simulink model "Q_4"  (Simulink 10.0)
settings: Solver=VariableStepAuto  StartTime=0.0  StopTime=10.0  RelTol=1e-3
settings Model: Creator=amirhosein  LastModifiedBy=amirhosein
settings DataIOCC: SaveFormat=Dataset  ReturnWorkspaceOutputs=on
settings OptimizationCC: LifeSpan=auto
settings DebuggingCC: UnderspecifiedInitializationDetection=Simplified  MergeDetectMultiDrivingBlocksExec=error  SFUnexpectedBacktrackingDiag=error  SFNoUnconditionalDefaultTransitionDiag=error  SFExecutionAtInitializationDiag=warning  ArithmeticOperatorsInVariantConditions=error
settings HardwareCC: ProdBitPerPointer=64  ProdBitPerSizeT=64  ProdBitPerPtrDiffT=64  ProdLargestAtomicFloat=Float  ProdIntDivRoundTo=Zero  ProdEndianess=LittleEndian  ProdWordSize=64  ProdHWDeviceType=Intel->x86-64 (Windows64)
settings ModelReferenceCC: PropagateSignalLabelsOutOfModel=on
settings SFSimCC: SimUseLocalCustomCode=on  CustomCodeUndefinedFunction=FilterOut
settings RTWCC: RTWUseLocalCustomCode=on
settings CodeAppCC: StateflowObjectComments=off
settings GRTTargetCC: TargetLangStandard=C99 (ISO)  CombineOutputUpdateFcns=on  GRTInterface=off
settings ConfigComp: CovMetricSettings=dwe  CovHtmlReporting=off  CovSaveCumulativeToWorkspaceVar=off  CovSaveSingleToWorkspaceVar=off

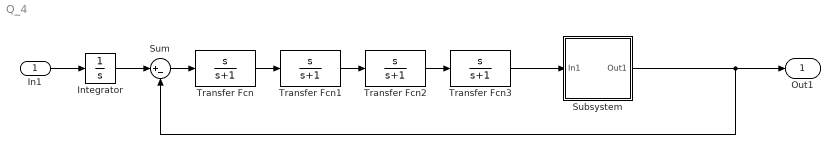
== system Q_4 ==
  In1 : Inport
  Integrator : Integrator
  Subsystem : Subsystem
  Sum : Sum  Inputs=|+-
  Transfer Fcn{,1..3} (4 alike) : TransferFcn  Numerator=[1 0]  Denominator=[1 1]
  Out1 : Outport
  wires:
  Integrator/1 -> Sum/1
  Transfer Fcn1/1 -> Transfer Fcn2/1
  Transfer Fcn/1 -> Transfer Fcn1/1
  Transfer Fcn2/1 -> Transfer Fcn3/1
  Sum/1 -> Transfer Fcn/1
  In1/1 -> Integrator/1
  Subsystem/1(Out1) -> Out1/1, Sum/2
  Transfer Fcn3/1 -> Subsystem/1(In1)

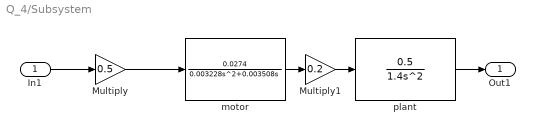
== system Q_4/Subsystem ==
  In1 : Inport
  Multiply : Gain  Gain=0.5
  Multiply1 : Gain  Gain=0.2
  motor : TransferFcn  Numerator=[0.0274]  Denominator=[0.003228 0.003508 0]
  plant : TransferFcn  Numerator=[0.5]  Denominator=[1.4 0 0 ]
  Out1 : Outport
  wires:
  Multiply1/1 -> plant/1
  motor/1 -> Multiply1/1
  Multiply/1 -> motor/1
  In1/1 -> Multiply/1
  plant/1 -> Out1/1
